simulink model "Model_3"  (R2020b)
settings: Solver=VariableStepAuto  StartTime=0.0  StopTime=10.0  RelTol=1e-3
undefined symbols (not defined in the file): R, vo
settings Model: Creator=Akarsh  LastModifiedBy=Akarsh

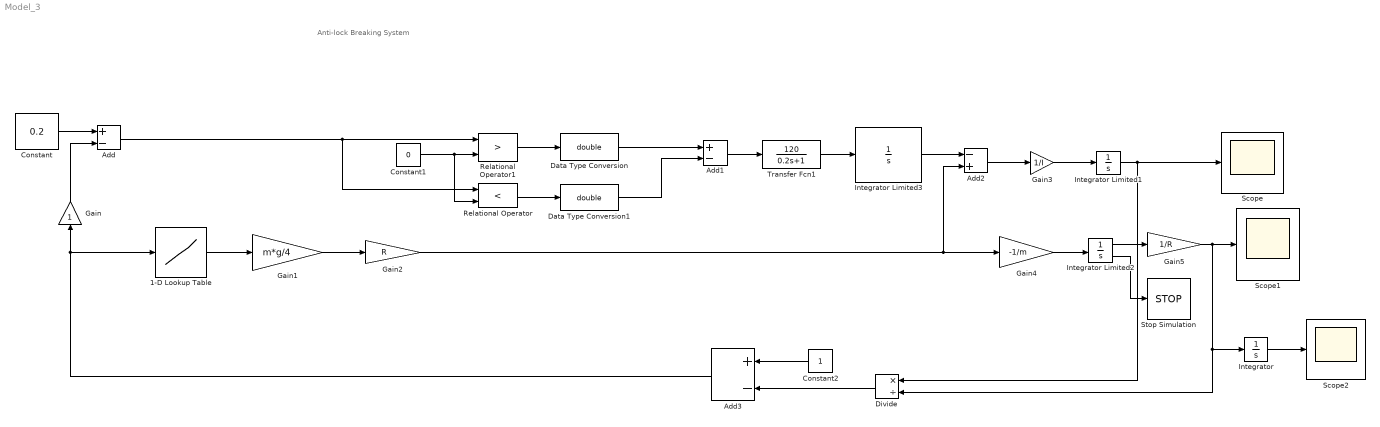
== system Model_3 ==
  note: Anti-lock Breaking System
  1-D Lookup Table : Lookup_n-D  NumberOfTableDimensions=1  BreakpointsForDimension1=[-5:5]  Table=tanh([-5:5])  InternalRulePriority=Speed  RndMeth=Simplest  InputSameDT=on
  Add : Sum  Inputs=+-
  Add1 : Sum  Inputs=+-
  Add2 : Sum  Inputs=-+
  Add3 : Sum  Inputs=+-
  Constant : Constant  Value=0.2
  Constant1 : Constant  Value=0
  Constant2 : Constant
  Data Type Conversion : DataTypeConversion  OutDataTypeStr=double  RndMeth=Zero
  Data Type Conversion1 : DataTypeConversion  OutDataTypeStr=double  RndMeth=Zero
  Divide : Product  Inputs=*/
  Gain : Gain
  Gain1 : Gain  Gain=m*g/4  mask{m=80, g=9.8}
  Gain2 : Gain  Gain=R  mask{R=1.5}
  Gain3 : Gain  Gain=1/I  mask{I=5}
  Gain4 : Gain  Gain=-1/m  mask{m=80}
  Gain5 : Gain  Gain=1/R  mask{R=1.5}
  Integrator : Integrator
  Integrator Limited1 : Integrator  InitialCondition=vo/R  LimitOutput=on  UpperSaturationLimit=1000  LowerSaturationLimit=0
  Integrator Limited2 : Integrator  InitialCondition=vo  LimitOutput=on  UpperSaturationLimit=1000  LowerSaturationLimit=0  ShowSaturationPort=on
  Integrator Limited3 : Integrator  LimitOutput=on  UpperSaturationLimit=1000  LowerSaturationLimit=0
  Relational Operator : RelationalOperator  Operator=<  OutDataTypeStr=boolean  RndMeth=Simplest
  Relational Operator1 : RelationalOperator  Operator=>  OutDataTypeStr=boolean  RndMeth=Simplest
  Scope : Scope
  Scope1 : Scope
  Scope2 : Scope
  Stop Simulation : Stop
  Transfer Fcn1 : TransferFcn  Numerator=120  Denominator=[0.2 1]
  wires:
  Constant/1 -> Add/1
  Gain/1 -> Add/2
  Add3/1 -> 1-D Lookup Table/1, Gain/1
  1-D Lookup Table/1 -> Gain1/1
  Gain1/1 -> Gain2/1
  Constant1/1 -> Relational Operator1/2, Relational Operator/2
  Add/1 -> Relational Operator1/1, Relational Operator/1
  Relational Operator1/1 -> Data Type Conversion/1
  Relational Operator/1 -> Data Type Conversion1/1
  Data Type Conversion/1 -> Add1/1
  Data Type Conversion1/1 -> Add1/2
  Add1/1 -> Transfer Fcn1/1
  Transfer Fcn1/1 -> Integrator Limited3/1
  Integrator Limited3/1 -> Add2/1
  Gain2/1 -> Gain4/1, Add2/2
  Add2/1 -> Gain3/1
  Gain3/1 -> Integrator Limited1/1
  Integrator Limited1/1 -> Divide/1, Scope/1
  Gain4/1 -> Integrator Limited2/1
  Integrator Limited2/1 -> Gain5/1
  Gain5/1 -> Divide/2, Integrator/1, Scope1/1
  Integrator Limited2/2 -> Stop Simulation/1
  Integrator/1 -> Scope2/1
  Divide/1 -> Add3/2
  Constant2/1 -> Add3/1
